simulink model "project2_week3"  (R2020b)
settings: Solver=VariableStepAuto  StartTime=0.0  StopTime=10.0  RelTol=1e-3
settings Model: Creator=RASIKA MALGI  LastModifiedBy=RASIKA MALGI

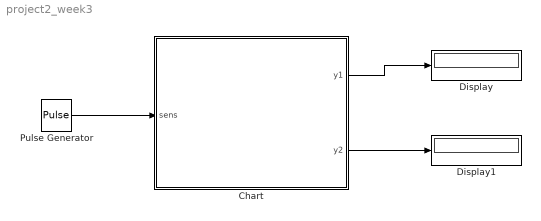
== system project2_week3 ==
  Chart : Stateflow chart  TreatAsAtomicUnit=on
  Display : Display
  Display1 : Display
  Pulse Generator : DiscretePulseGenerator  PulseType=Time based  Period=10  PulseWidth=5
  wires:
  Pulse Generator/1 -> Chart/1(sens)
  Chart/2(y2) -> Display1/1
  Chart/1(y1) -> Display/1

== stateflow chart project2_week3/Chart ==
  state Stop
    y1=RED;
    y2=GREEN;
  state Stop_for_traffic
    y1=RED;
    y2=GREEN;
  state Stop_to_go
    y1=RED;
    y2=YELLOW;
  state Go_to_stop
    y1=YELLOW;
    y2=RED;
  state Go
    y1=GREEN;
    y2=RED;
  (default) -> Stop
  Stop -> Stop_for_traffic : after(20,tick)
  Stop_for_traffic -> Stop_to_go : [sens]
  Go_to_stop -> Stop : after(3,tick)
  Stop_to_go -> Go : after(3,tick)
  Go -> Go_to_stop : after(10,tick)
  data: sens input; y1 output; y2 output; GREEN constant double =3; RED constant double =1; YELLOW constant double =2
